simulink model "simulink_fuzzy"  (R2021b)
settings: Solver=VariableStepAuto  StartTime=0.0  StopTime=50.0  RelTol=1e-3
libraries: fuzblock x1
settings Model: Creator=THANH DAT  LastModifiedBy=THANH DAT

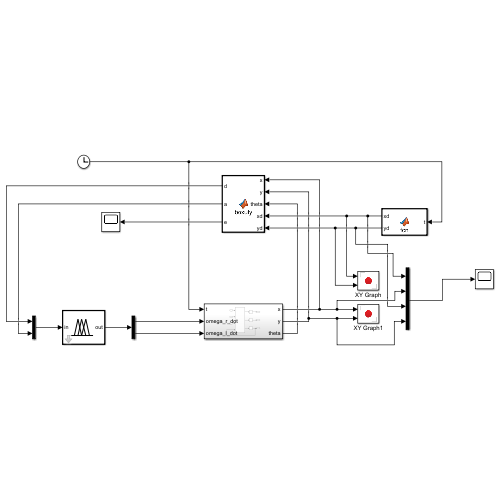
[thumbnail: Simulink's stored preview of the top-level diagram]
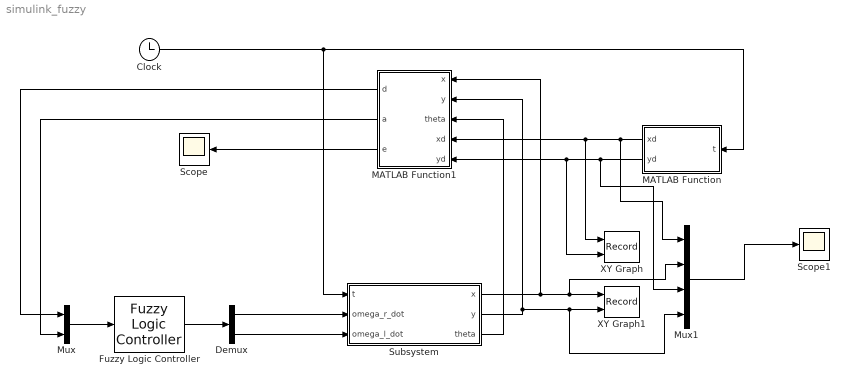
== system simulink_fuzzy ==
  Clock : Clock
  Demux : Demux  Outputs=2
  Fuzzy Logic Controller : fuzblock/Fuzzy Logic  Controller  FIS='fuzzy_wmr_func'  OutputSampleNumber=101  DataType=double  FuzzifiedInputs=off  RuleFiringStrengths=off  RuleOutputs=off  AggregatedOutputs=off  SimulateUsing=Interpreted execution  OutOfRangeInputValueMessage=warning  NoRuleFiredMessage=warning  EmptyOutputFuzzySetMessage=warning
  MATLAB Function : MATLAB Function  TreatAsAtomicUnit=on
  MATLAB Function1 : MATLAB Function  TreatAsAtomicUnit=on
  Mux : Mux  Inputs=2
  Mux1 : Mux
  Scope : Scope
  Scope1 : Scope
  Subsystem : Subsystem
  XY Graph : Record  FileSettingsInternal="{\"entries\":[{\"content\":{\"excelSettings\":{\"content\":{},\"type\":\"Streamout.ExcelSettings\"}},\"type\":\"Streamout.FileSettingStorage\",\"uuid\":\"83b2480a-f607-47d0-8db9-3262f1c91061\"}],\"packageUris\":[\"http://schema.mathworks.com/mf0/streamout_blocks/R2020a\"],\"version\":\"1.0\"}"  Layout=[1 1]  SignalsInternal="{\"entries\":[{\"content\":{\"signals\":[{\"content\":{\"blockPath\":[\"simulink_fuzzy/XY Graph\"],\"channel\":[],\"dimensions\":[1],\"domain\":\"simulink_fuzzy/XY Graph\",\"lineColor\":\"#a2142f\",\"plots\":[1],\"port\":1,\"sid\":[\"\"],\"signalID\":75221,\"signalName\":\"MATLAB Function:1\"},\"type\":\"RecordBlkView.Signal\",\"uuid\":\"640e0465-435a-46d4-80c4-0aea7fbbff71\"},{\"content\":{\"blockPath\":[\"simulink_fuzzy/XY Graph\"],\"channel\":[],\"dimensions\":[1],\"domain\":\"simulink_fuzzy/XY Graph\",\"lineColor\":\"#139fff\",\"plots\":[1],\"port\":2,\"sid\":[\"\"],\"signalID\":75225,\"signalName\":\"MATLAB Function:2\"},\"type\":\"RecordBlkView.Signal\",\"uuid\":\"3fd2994c-0382-488e-9bfb-b67706cb4f47\"}]},\"type\":\"RecordBlkView.InputSignals\",\"uuid\":\"26c28319-cd72-488b-bde7-5ad99c7d05a2\"}],\"packageUris\":[\"http://schema.mathworks.com/mf0/streamout_blocks/R2020a\"],\"version\":\"1.0\"}"  VisualizationBindings="{\"xyplotplugin\":{\"info\":[{\"series\":[{\"bindingParametersList\":[{\"parameter\":\"X-Axis\",\"signalID\":75221,\"signalName\":\"MATLAB Function:1\"},{\"parameter\":\"Y-Axis\",\"signalID\":75225,\"signalName\":\"MATLAB Function:2\"}],\"seriesID\":49733}],\"subplotID\":1}]}}"  CompatibilityTag=XY
  XY Graph1 : Record  FileSettingsInternal="{\"entries\":[{\"content\":{\"excelSettings\":{\"content\":{},\"type\":\"Streamout.ExcelSettings\"}},\"type\":\"Streamout.FileSettingStorage\",\"uuid\":\"73105d5f-67e9-499b-ad00-84f455f31b5f\"}],\"packageUris\":[\"http://schema.mathworks.com/mf0/streamout_blocks/R2020a\"],\"version\":\"1.0\"}"  Layout=[1 1]  SignalsInternal="{\"entries\":[{\"content\":{\"signals\":[{\"content\":{\"blockPath\":[\"simulink_fuzzy/XY Graph1\"],\"channel\":[],\"dimensions\":[1],\"domain\":\"simulink_fuzzy/XY Graph1\",\"lineColor\":\"#a2142f\",\"plots\":[1],\"port\":1,\"sid\":[\"\"],\"signalID\":75229,\"signalName\":\"Subsystem:1\"},\"type\":\"RecordBlkView.Signal\",\"uuid\":\"5111a881-2a90-47c5-af5a-38cb0a819e19\"},{\"content\":{\"blockPath\":[\"simulink_fuzzy/XY Graph1\"],\"channel\":[],\"dimensions\":[1],\"domain\":\"simulink_fuzzy/XY Graph1\",\"lineColor\":\"#139fff\",\"plots\":[1],\"port\":2,\"sid\":[\"\"],\"signalID\":75233,\"signalName\":\"Subsystem:2\"},\"type\":\"RecordBlkView.Signal\",\"uuid\":\"48a7a6f8-0524-4434-b156-59e61b400143\"}]},\"type\":\"RecordBlkView.InputSignals\",\"uuid\":\"7f577cbe-44bc-4aba-aef0-64430aa848e7\"}],\"packageUris\":[\"http://schema.mathworks.com/mf0/streamout_blocks/R2020a\"],\"version\":\"1.0\"}"  VisualizationBindings="{\"xyplotplugin\":{\"info\":[{\"series\":[{\"bindingParametersList\":[{\"parameter\":\"X-Axis\",\"signalID\":75229,\"signalName\":\"Subsystem:1\"},{\"parameter\":\"Y-Axis\",\"signalID\":75233,\"signalName\":\"Subsystem:2\"}],\"seriesID\":20195}],\"subplotID\":1}]}}"  CompatibilityTag=XY
  wires:
  Fuzzy Logic Controller/1 -> Demux/1
  Mux/1 -> Fuzzy Logic Controller/1
  Demux/1 -> Subsystem/2(omega_r_dot)
  Demux/2 -> Subsystem/3(omega_l_dot)
  Clock/1 -> Subsystem/1(t), MATLAB Function/1(t)
  Subsystem/1(x) -> Mux1/2, XY Graph1/1, MATLAB Function1/1(x)
  Subsystem/2(y) -> Mux1/4, XY Graph1/2, MATLAB Function1/2(y)
  Subsystem/3(theta) -> MATLAB Function1/3(theta)
  MATLAB Function1/1(d) -> Mux/1
  MATLAB Function1/2(a) -> Mux/2
  MATLAB Function/1(xd) -> Mux1/1, MATLAB Function1/4(xd), XY Graph/1
  MATLAB Function/2(yd) -> Mux1/3, XY Graph/2, MATLAB Function1/5(yd)
  MATLAB Function1/3(e) -> Scope/1
  Mux1/1 -> Scope1/1

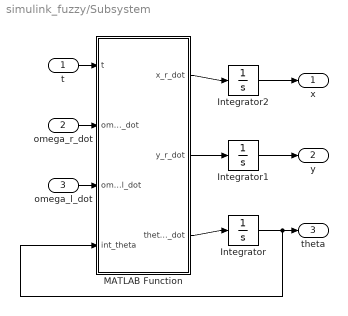
== system simulink_fuzzy/Subsystem ==
  t : Inport
  omega_r_dot : Inport  Port=2
  omega_l_dot : Inport  Port=3
  Integrator : Integrator
  Integrator1 : Integrator
  Integrator2 : Integrator
  MATLAB Function : MATLAB Function  TreatAsAtomicUnit=on
  x : Outport
  y : Outport  Port=2
  theta : Outport  Port=3
  wires:
  Integrator/1 -> theta/1, MATLAB Function/4(int_theta)
  MATLAB Function/1(x_r_dot) -> Integrator2/1
  omega_l_dot/1 -> MATLAB Function/3(omega_l_dot)
  Integrator2/1 -> x/1
  MATLAB Function/2(y_r_dot) -> Integrator1/1
  MATLAB Function/3(theta_dot) -> Integrator/1
  omega_r_dot/1 -> MATLAB Function/2(omega_r_dot)
  t/1 -> MATLAB Function/1(t)
  Integrator1/1 -> y/1

== matlab function simulink_fuzzy/MATLAB Function1 ==
  data: x input; d output; y input; theta input; xd input; yd input; a output; e output
function [d,a,e] = boxuly(x,y,theta,xd,yd)

dx = xd-x;
dy = yd-y;
d=sqrt(dx^2+dy^2);
if(d>5)
    d = 4.99;
end
thetad = atan2(dy,dx);
a = thetad - theta; 
e = dx;

== matlab function simulink_fuzzy/Subsystem/MATLAB Function ==
  data: t input; x_r_dot output; omega_r_dot input; omega_l_dot input; int_theta input; y_r_dot output; theta_dot output
function [x_r_dot, y_r_dot, theta_dot] = kinematic(t, omega_r_dot, omega_l_dot, int_theta)
%Declaration
r = 0.15; %radius of the wheel
b = 0.3;  %radius of the wheel shaft
a = 0.2; %distance between the R and PG
mG = 10; %weight of the platform
mW = 2; %weight of each wheel
IG = 4; %inertial moment of the platform
ID = 0.05; %inertial moment of each wheel
IW = 0.1;  %inertial moment of each wheel

%Variable
gamma_r_dot = 0; 
gamma_l_dot = 0;
eta_dot =0;
%Kinematic
sigma = r*(omega_r_dot + omega_l_dot)/2 + (gamma_r_dot + gamma_l_dot)/2;          %u foward velocity 
eta = eta_dot;                                                                    %v 
omega = r*(omega_r_dot - omega_l_dot)/(2*b) + (gamma_r_dot - gamma_l_dot)/(2*b);  %r

theta = int_theta;
theta_dot = omega; 

Jacobi = [cos(theta), -sin(theta), 0;
     sin(theta), cos(theta), 0;
     0, 0, 1;];

T = [sigma;
    eta;
    omega;];

V = Jacobi*T; 
x_r_dot = V(1,1);
y_r_dot = V(2,1);

== matlab function simulink_fuzzy/MATLAB Function ==
  data: t input; xd output; yd output
function [xd, yd] = fcn(t)

yd = sin(0.5*t)+0.5*t + 1; 
xd = -t; 
% yd = 13*cos((pi/20)*t)-5*cos((2*pi/20)*t)-2*cos((3*pi/20)*t)-cos((pi/20)*t);
% xd = 12*sin((pi/20)*t)-4*sin((pi/20)*t);
